simulink model "Sim_Forcing_003h_expe_infra2"  (Simulink 7.4)
settings: Solver=FixedStepDiscrete  StartTime=0.0  StopTime=inf  FixedStep=0.004  RelTol=1e-3
undefined symbols (not defined in the file or in its folder): DiscIntNeverNeededParam
libraries: simulink x42, gt_rt_lib x30, xpcutilitieslib x9, xpclib x2, dspswit3 x1
(part 2 of 5)

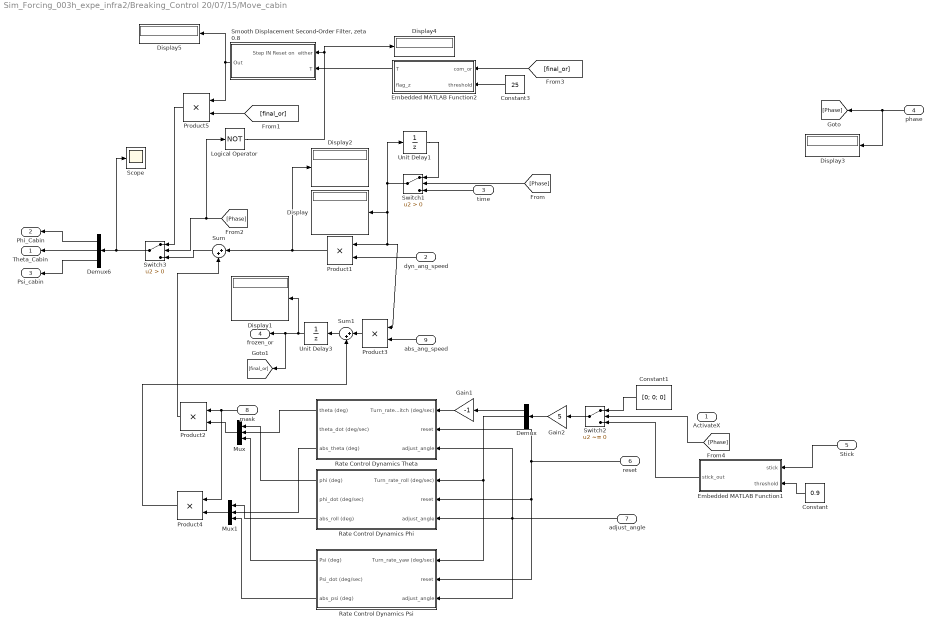
== system Sim_Forcing_003h_expe_infra2/Breaking_Control 20/07/15/Move_cabin ==
  ActivateX : Inport
  dyn_ang_speed : Inport  Port=2
  time : Inport  Port=3
  phase : Inport  Port=4
  Stick : Inport  Port=5
  reset : Inport  Port=6
  adjust_angle : Inport  Port=7
  mask : Inport  Port=8
  abs_ang_speed : Inport  Port=9
  Constant : Constant  Value=0.9  OutDataType=fixdt(1, 16)  OutScaling=2^0
  Constant1 : Constant  Value=[0; 0; 0]  OutDataType=fixdt(1, 16)  OutScaling=2^0
  Constant3 : Constant  Value=25  OutDataType=fixdt(1, 16)  OutScaling=2^0  SampleTime=-1
  Demux : Demux  Outputs=3
  Demux6 : Demux  Outputs=3
  Display{,1..5} (6 alike) : Display
  Embedded MATLAB Function1 : Stateflow chart
  Embedded MATLAB Function2 : Stateflow chart
  Gain1 : Gain  Gain=-1  ParameterDataType=fixdt(1, 16)  ParameterScaling=2^0  OutDataType=fixdt(1, 16)  OutScaling=2^0
  Gain2 : Gain  Gain=5  ParameterDataType=fixdt(1, 16)  ParameterScaling=2^0  OutDataType=fixdt(1, 16)  OutScaling=2^0
  Logical Operator : Logic  Operator=NOT  AllPortsSameDT=off  OutDataTypeMode=boolean  LogicDataType=fixdt(0, 8)  OutDataTypeStr=boolean
  Mux : Mux  Inputs=3
  Mux1 : Mux  Inputs=3
  Product{1..5} (5 alike) : Product  OutDataType=fixdt(1, 16)  OutScaling=2^0  RndMeth=Zero
  Rate Control Dynamics Phi : Subsystem
  Rate Control Dynamics Psi : Subsystem
  Rate Control Dynamics Theta : Subsystem
  Scope : Scope
      settings: TimeRange=10  YMin=0  YMax=4.5e-033  SaveName=ScopeData2
  "Smooth Displacement Second-Order Filter, zeta 0.8" : Subsystem
  Sum : Sum  Inputs=|++  OutDataType=fixdt(1, 16)  OutScaling=2^0
  Sum1 : Sum  Inputs=|++  OutDataType=fixdt(1, 16)  OutScaling=2^0
  Switch1 : Switch  Criteria=u2 > Threshold  OutDataType=fixdt(1, 16)  OutScaling=2^0
  Switch2 : Switch  Criteria=u2 ~= 0  OutDataType=fixdt(1, 16)  OutScaling=2^0
  Switch3 : Switch  Criteria=u2 > Threshold  OutDataType=fixdt(1, 16)  OutScaling=2^0
  Unit Delay1 : UnitDelay  X0=[0 0 0]  SampleTime=-1
  Unit Delay3 : UnitDelay  X0=[0 0 0]  SampleTime=-1
  Theta_Cabin : Outport
  Phi_Cabin : Outport  Port=2
  Psi_cabin : Outport  Port=3
  frozen_or : Outport  Port=4
  wires:
  Demux6/3 -> Psi_cabin/1
  Switch1/1 -> Unit Delay1/1, Display/1, Product1/1, Product3/1
  time/1 -> Switch1/3
  Unit Delay1/1 -> Switch1/1
  Gain2/1 -> Demux/1
  Demux/1 -> Gain1/1
  Demux/2 -> Rate Control Dynamics Phi/1(Turn_rate_roll (deg/sec)), Rate Control Dynamics Psi/1(Turn_rate_yaw (deg/sec))
  Product1/1 -> Display2/1, Sum/1
  reset/1 -> Rate Control Dynamics Theta/2(reset), Rate Control Dynamics Phi/2(reset), Rate Control Dynamics Psi/2(reset)
  adjust_angle/1 -> Rate Control Dynamics Phi/3(adjust_angle), Rate Control Dynamics Theta/3(adjust_angle), Rate Control Dynamics Psi/3(adjust_angle)
  Rate Control Dynamics Theta/1(theta (deg)) -> Mux/2
  Rate Control Dynamics Phi/1(phi (deg)) -> Mux/1
  Mux/1 -> Product2/2
  mask/1 -> Product2/1, Product4/1
  Demux6/1 -> Phi_Cabin/1
  Demux6/2 -> Theta_Cabin/1
  Gain1/1 -> Rate Control Dynamics Theta/1(Turn_rate_pitch (deg/sec))
  Switch2/1 -> Gain2/1
  Rate Control Dynamics Psi/1(Psi (deg)) -> Mux/3
  dyn_ang_speed/1 -> Product1/2
  phase/1 -> [Phase], Display3/1
  [Phase] -> Switch1/2
  Product2/1 -> Sum/2
  Unit Delay3/1 -> Display1/1, frozen_or/1, [final_or]
  Sum1/1 -> Unit Delay3/1
  Product3/1 -> Sum1/1
  abs_ang_speed/1 -> Product3/2
  Mux1/1 -> Product4/2
  Rate Control Dynamics Theta/3(abs_theta (deg)) -> Mux1/2
  Product4/1 -> Sum1/2
  Rate Control Dynamics Phi/3(abs_roll (deg)) -> Mux1/1
  Rate Control Dynamics Psi/3(abs_psi (deg)) -> Mux1/3
  [final_or] -> Product5/2
  "Smooth Displacement Second-Order Filter, zeta 0.8"/1(Out) -> Product5/1, Display5/1
  Switch3/1 -> Demux6/1, Scope/1
  Sum/1 -> Switch3/3
  Product5/1 -> Switch3/1
  [Phase] -> Switch3/2, Logical Operator/1
  Logical Operator/1 -> "Smooth Displacement Second-Order Filter, zeta 0.8"/1(Step IN Reset on  either), Display4/1
  Constant3/1 -> Embedded MATLAB Function2/2(threshold)
  [final_or] -> Embedded MATLAB Function2/1(com_or)
  Embedded MATLAB Function2/1(T) -> "Smooth Displacement Second-Order Filter, zeta 0.8"/2(T)
  Stick/1 -> Embedded MATLAB Function1/1(stick)
  Constant/1 -> Embedded MATLAB Function1/2(threshold)
  [Phase] -> Switch2/2
  Constant1/1 -> Switch2/1
  Embedded MATLAB Function1/1(stick_out) -> Switch2/3

== system Sim_Forcing_003h_expe_infra2/Breaking_Control 20/07/15/Save_data1 ==
  note: we take delay_in + delay_out. We assume it remains cst
  count : Inport  OutDataType=fixdt(1, 16)  OutScaling=2^0
  delay : Inport  Port=2  OutDataType=fixdt(1, 16)  OutScaling=2^0
  Actual_orientation : Inport  Port=3  OutDataType=fixdt(1, 16)  OutScaling=2^0
  com_orientation : Inport  Port=4  OutDataType=fixdt(1, 16)  OutScaling=2^0
  target_ang_speed : Inport  Port=5  OutDataType=fixdt(1, 16)  OutScaling=2^0
  time : Inport  Port=6  OutDataType=fixdt(1, 16)  OutScaling=2^0
  IsinRestPhase : Inport  Port=7  OutDataType=fixdt(1, 16)  OutScaling=2^0
  vis_cond : Inport  Port=8  OutDataType=fixdt(1, 16)  OutScaling=2^0
  Enable : EnablePort  ShowOutputPort=on
  6_DOF Visual Cab 12/06/15 : Subsystem
  Gain : Gain  ParameterDataType=fixdt(1, 16)  ParameterScaling=2^0  OutDataType=fixdt(1, 16)  OutScaling=2^0
  act_or : Display
  or : Display
  wires:
  delay/1 -> Gain/1
  com_orientation/1 -> or/1, 6_DOF Visual Cab 12/06/15/2(Com_or)
  count/1 -> [Cnt]
  time/1 -> [time]
  [time] -> 6_DOF Visual Cab 12/06/15/1(time)
  [targ_ang_speed] -> 6_DOF Visual Cab 12/06/15/5(targ_ang_speed)
  Gain/1 -> 6_DOF Visual Cab 12/06/15/6(delay)
  [reset] -> 6_DOF Visual Cab 12/06/15/8(reset)
  IsinRestPhase/1 -> [RestPhase]
  [RestPhase] -> 6_DOF Visual Cab 12/06/15/7(IsinRestPhase2)
  [Cnt] -> 6_DOF Visual Cab 12/06/15/4(cnt)
  vis_cond/1 -> 6_DOF Visual Cab 12/06/15/3(Vis_cond)
  target_ang_speed/1 -> [targ_ang_speed]
  Actual_orientation/1 -> 6_DOF Visual Cab 12/06/15/9(act_or), act_or/1

== system Sim_Forcing_003h_expe_infra2/Breaking_Control 20/07/15/Send_to_noise_node ==
  note: Send to beat node
  trigger_noise : Inport
  "Byte Packing " : xpcutilitieslib/Byte Packing   MaskPackedDataType=uint8  MaskUnpackedDataTypes={'single'}  MaskAlignment=1
  Constant2 : Constant  Value=9350  OutDataTypeMode=uint16  OutDataType=fixdt(1, 16)  OutScaling=2^0  OutDataTypeStr=uint16
  Constant3 : Constant  Value=4  OutDataTypeMode=uint32  OutDataType=fixdt(1, 16)  OutScaling=2^0  OutDataTypeStr=uint32
  Data Type Conversion : DataTypeConversion  OutDataTypeMode=single  OutDataType=fixdt(1, 16)  OutScaling=2^0  OutDataTypeStr=single
  Display : Display
  GT-RT UDP  Write : gt_rt_lib/GT-RT UDP  Controller  uri='gtp://localhost/udp?port=9350'
  GT-RT UDP TX : gt_rt_lib/GT-RT UDP TX  uri='gtp://localhost/udp?port=9350'  hostname='192.168.102.75'
  Write Error : Display
  wires:
  Constant2/1 -> GT-RT UDP TX/2
  GT-RT UDP TX/1 -> Write Error/1
  Data Type Conversion/1 -> "Byte Packing "/1
  trigger_noise/1 -> Data Type Conversion/1, Display/1
  Constant3/1 -> GT-RT UDP TX/4
  "Byte Packing "/1 -> GT-RT UDP TX/3

== system Sim_Forcing_003h_expe_infra2/Breaking_Control 20/07/15/Smooth Displacement Second-Order Filter, zeta 0.8 ==
  Step IN Reset on  either : Inport
  T : Inport  Port=2  OutDataType=fixdt(1, 16)  OutScaling=2^0
  (zeta*T_transfer)/pi : Gain  Gain=0.8/pi  ParameterDataType=fixdt(1, 16)  ParameterScaling=2^0  OutDataType=fixdt(1, 16)  OutScaling=2^0
  4*zeta*pi : Gain  Gain=3.2*pi  ParameterDataType=fixdt(1, 16)  ParameterScaling=2^0  OutDataType=fixdt(1, 16)  OutScaling=2^0
  4*zeta*pi/T_transfer /s : DiscreteIntegrator  gainval=1  ExternalReset=either  InitialConditionSource=external  SampleTime=0.004  OutDataType=fixdt(1, 16)  OutScaling=2^0  ICPrevOutput=DiscIntNeverNeededParam  ICPrevScaledInput=DiscIntNeverNeededParam
  Discrete Derivative : simulink/Discrete/Discrete Derivative  SystemSampleTime=-1  gainval=1.0  ICPrevScaledInput=0.0  OutMin=[]  OutMax=[]  OutDataType=fixdt(1, 16)  OutScaling=2^-10  DoSatur=off
  Divide : Product  Inputs=*/  OutDataType=fixdt(1, 16)  OutScaling=2^-10
  Divide1 : Product  Inputs=*/  OutDataType=fixdt(1, 16)  OutScaling=2^-10
  For saving position  and velocity until after switchover : UnitDelay  SampleTime=-1
  Product : Product  OutDataType=fixdt(1, 16)  OutScaling=2^0  RndMeth=Zero
  Sum1 : Sum  Inputs=|+-  OutDataType=fixdt(1, 16)  OutScaling=2^0
  Sum2 : Sum  Inputs=-+|  OutDataType=fixdt(1, 16)  OutScaling=2^0
  pi/(zeta*T_transfer)/s : DiscreteIntegrator  gainval=1  ExternalReset=either  InitialConditionSource=external  SampleTime=0.004  OutDataType=fixdt(1, 16)  OutScaling=2^0  ICPrevOutput=DiscIntNeverNeededParam  ICPrevScaledInput=DiscIntNeverNeededParam
  pi/zeta : Gain  Gain=pi/0.8  ParameterDataType=fixdt(1, 16)  ParameterScaling=2^0  OutDataType=fixdt(1, 16)  OutScaling=2^0
  Out : Outport
  wires:
  Discrete Derivative/1 -> Product/2
  Product/1 -> (zeta*T_transfer)/pi/1
  Divide/1 -> 4*zeta*pi/1
  Divide1/1 -> pi/zeta/1
  pi/zeta/1 -> pi/(zeta*T_transfer)/s/1
  pi/(zeta*T_transfer)/s/1 -> Sum2/1, Out/1, For saving position  and velocity until after switchover/1
  4*zeta*pi/T_transfer /s/1 -> Divide1/1, Sum1/2
  Sum1/1 -> Divide/1
  4*zeta*pi/1 -> 4*zeta*pi/T_transfer /s/1
  T/1 -> [T]
  Step IN Reset on  either/1 -> [Step], Sum2/2
  [Step] -> 4*zeta*pi/T_transfer /s/2
  [Step] -> pi/(zeta*T_transfer)/s/2
  [T] -> Divide/2
  For saving position  and velocity until after switchover/1 -> Discrete Derivative/1, pi/(zeta*T_transfer)/s/3
  [T] -> Product/1
  (zeta*T_transfer)/pi/1 -> 4*zeta*pi/T_transfer /s/3
  [T] -> Divide1/2
  Sum2/1 -> Sum1/1

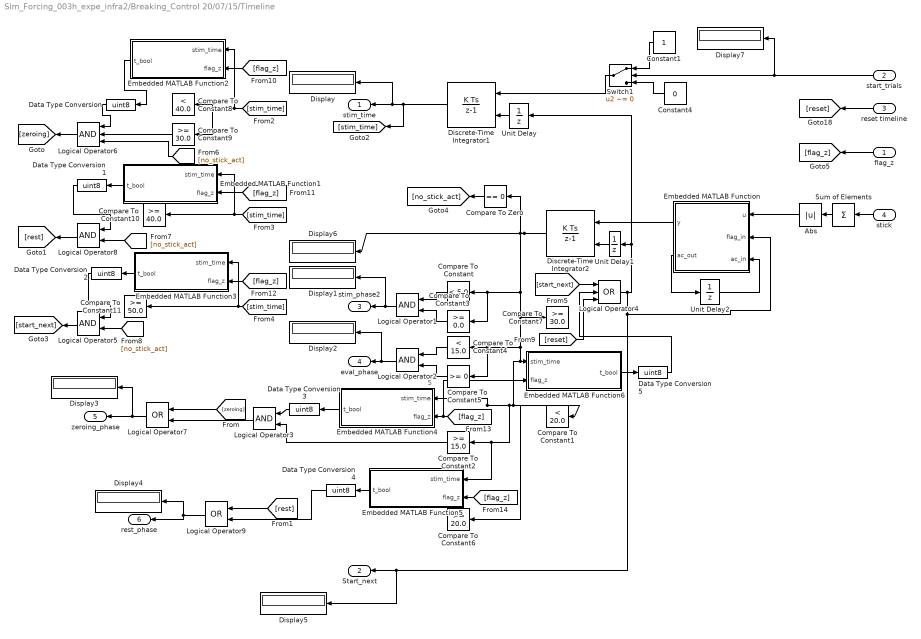
== system Sim_Forcing_003h_expe_infra2/Breaking_Control 20/07/15/Timeline ==
  note: 5
  flag_z : Inport  PortDimensions=1
  start_trials : Inport  Port=2  PortDimensions=1
  reset timeline : Inport  Port=3  PortDimensions=1
  stick : Inport  Port=4
  Abs : Abs  OutDataType=fixdt(1, 16)  OutScaling=2^0
  Compare To Constant : simulink/Logic and Bit Operations/Compare To Constant  SystemSampleTime=-1  relop=<  const=5.0  LogicOutDataTypeMode=uint8
  Compare To Constant1 : simulink/Logic and Bit Operations/Compare To Constant  SystemSampleTime=-1  relop=<  const=20.0  LogicOutDataTypeMode=uint8
  Compare To Constant10 : simulink/Logic and Bit Operations/Compare To Constant  SystemSampleTime=-1  relop=>=  const=40.0  LogicOutDataTypeMode=uint8
  Compare To Constant11 : simulink/Logic and Bit Operations/Compare To Constant  SystemSampleTime=-1  relop=>=  const=50.0  LogicOutDataTypeMode=uint8
  Compare To Constant2 : simulink/Logic and Bit Operations/Compare To Constant  SystemSampleTime=-1  relop=>=  const=15.0  LogicOutDataTypeMode=uint8
  Compare To Constant3 : simulink/Logic and Bit Operations/Compare To Constant  SystemSampleTime=-1  relop=>=  const=0.0  LogicOutDataTypeMode=uint8
  Compare To Constant4 : simulink/Logic and Bit Operations/Compare To Constant  SystemSampleTime=-1  relop=<  const=15.0  LogicOutDataTypeMode=uint8
  Compare To Constant5 : simulink/Logic and Bit Operations/Compare To Constant  SystemSampleTime=-1  relop=>=  const=0  LogicOutDataTypeMode=uint8
  Compare To Constant6 : simulink/Logic and Bit Operations/Compare To Constant  SystemSampleTime=-1  relop=>=  const=20.0  LogicOutDataTypeMode=uint8
  Compare To Constant7 : simulink/Logic and Bit Operations/Compare To Constant  SystemSampleTime=-1  relop=>=  const=30.0  LogicOutDataTypeMode=uint8
  Compare To Constant8 : simulink/Logic and Bit Operations/Compare To Constant  SystemSampleTime=-1  relop=<  const=40.0  LogicOutDataTypeMode=uint8
  Compare To Constant9 : simulink/Logic and Bit Operations/Compare To Constant  SystemSampleTime=-1  relop=>=  const=30.0  LogicOutDataTypeMode=uint8
  Compare To Zero : simulink/Logic and Bit Operations/Compare To Zero  SystemSampleTime=-1  relop===  LogicOutDataTypeMode=uint8
  Constant1 : Constant  OutDataType=fixdt(1, 16)  OutScaling=2^0
  Constant4 : Constant  Value=0  OutDataType=fixdt(1, 16)  OutScaling=2^0
  Data Type Conversion{,1..5} (6 alike) : DataTypeConversion  OutDataTypeMode=uint8  OutDataType=fixdt(1, 16)  OutScaling=2^0  OutDataTypeStr=uint8
  Discrete-Time Integrator1 : DiscreteIntegrator  ExternalReset=rising  SampleTime=0.004  LimitOutput=on  UpperSaturationLimit=60  LowerSaturationLimit=0  ICPrevOutput=DiscIntNeverNeededParam  ICPrevScaledInput=DiscIntNeverNeededParam
  Discrete-Time Integrator2 : DiscreteIntegrator  ExternalReset=level  SampleTime=0.004  LimitOutput=on  UpperSaturationLimit=40  LowerSaturationLimit=0  ICPrevOutput=DiscIntNeverNeededParam  ICPrevScaledInput=DiscIntNeverNeededParam
  Display{,1..7} (8 alike) : Display
  Embedded MATLAB Function : Stateflow chart
  Embedded MATLAB Function1 : Stateflow chart
  Embedded MATLAB Function2 : Stateflow chart
  Embedded MATLAB Function3 : Stateflow chart
  Embedded MATLAB Function4 : Stateflow chart
  Embedded MATLAB Function5 : Stateflow chart
  Embedded MATLAB Function6 : Stateflow chart
  Logical Operator{1..3,5,8} (5 alike) : Logic  AllPortsSameDT=off  OutDataTypeMode=boolean  LogicDataType=fixdt(0, 8)  OutDataTypeStr=boolean
  Logical Operator4 : Logic  Operator=OR  Inputs=3  AllPortsSameDT=off  OutDataTypeMode=boolean  LogicDataType=fixdt(0, 8)  OutDataTypeStr=boolean
  Logical Operator6 : Logic  Inputs=3  AllPortsSameDT=off  OutDataTypeMode=boolean  LogicDataType=fixdt(0, 8)  OutDataTypeStr=boolean
  Logical Operator7 : Logic  Operator=OR  AllPortsSameDT=off  OutDataTypeMode=boolean  LogicDataType=fixdt(0, 8)  OutDataTypeStr=boolean
  Logical Operator9 : Logic  Operator=OR  AllPortsSameDT=off  OutDataTypeMode=boolean  LogicDataType=fixdt(0, 8)  OutDataTypeStr=boolean
  Sum of Elements : Sum  Inputs=+  OutDataType=fixdt(1, 16)  OutScaling=2^-10
  Switch1 : Switch  Criteria=u2 ~= 0  Threshold=0.2  OutDataType=fixdt(1, 16)  OutScaling=2^0
  Unit Delay : UnitDelay  SampleTime=-1
  Unit Delay1 : UnitDelay  SampleTime=-1
  Unit Delay2 : UnitDelay  SampleTime=-1
  stim_time : Outport  OutDataType=fixdt(1, 16)  OutScaling=2^0
  Start_next : Outport  Port=2  OutDataType=fixdt(1, 16)  OutScaling=2^0
  stim_phase2 : Outport  Port=3  OutDataType=fixdt(1, 16)  OutScaling=2^0
  eval_phase : Outport  Port=4  OutDataType=fixdt(1, 16)  OutScaling=2^0
  zeroing_phase : Outport  Port=5  OutDataType=fixdt(1, 16)  OutScaling=2^0
  rest_phase : Outport  Port=6  OutDataType=fixdt(1, 16)  OutScaling=2^0
  wires:
  Discrete-Time Integrator1/1 -> stim_time/1, Display/1, [stim_time]
  Embedded MATLAB Function/1(y) -> Discrete-Time Integrator2/1
  Discrete-Time Integrator2/1 -> Compare To Constant/1, Compare To Constant3/1, Compare To Constant4/1, Compare To Constant5/1, Compare To Constant1/1, Embedded MATLAB Function4/1(stim_time), Compare To Constant2/1, Embedded MATLAB Function5/1(stim_time), Compare To Constant6/1, Embedded MATLAB Function6/1(stim_time), Compare To Constant7/1, Display6/1, Compare To Zero/1
  Compare To Constant/1 -> Logical Operator1/1
  Compare To Constant3/1 -> Logical Operator1/2
  Logical Operator1/1 -> stim_phase2/1, Display1/1
  Compare To Constant4/1 -> Logical Operator2/1
  Compare To Constant5/1 -> Logical Operator2/2
  Logical Operator2/1 -> eval_phase/1, Display2/1
  Compare To Constant2/1 -> Logical Operator3/2
  Logical Operator3/1 -> Logical Operator7/2
  Logical Operator4/1 -> Start_next/1, Display5/1, Embedded MATLAB Function/2(flag_in), Unit Delay1/1, Unit Delay/1
  Constant1/1 -> Switch1/1
  Switch1/1 -> Discrete-Time Integrator1/1
  start_trials/1 -> Switch1/2, Display7/1
  Constant4/1 -> Switch1/3
  stick/1 -> Sum of Elements/1
  Unit Delay/1 -> Discrete-Time Integrator1/2
  Unit Delay1/1 -> Discrete-Time Integrator2/2
  Sum of Elements/1 -> Abs/1
  Abs/1 -> Embedded MATLAB Function/1(u)
  Embedded MATLAB Function/2(ac_out) -> Unit Delay2/1
  Unit Delay2/1 -> Embedded MATLAB Function/3(ac_in)
  Compare To Constant9/1 -> Logical Operator6/2
  Logical Operator7/1 -> zeroing_phase/1, Display3/1
  Logical Operator9/1 -> rest_phase/1, Display4/1
  Logical Operator6/1 -> [zeroing]
  [zeroing] -> Logical Operator7/1
  Logical Operator8/1 -> [rest]
  [rest] -> Logical Operator9/1
  [stim_time] -> Compare To Constant8/1, Compare To Constant9/1, Embedded MATLAB Function2/1(stim_time)
  [stim_time] -> Compare To Constant10/1, Embedded MATLAB Function1/1(stim_time)
  [stim_time] -> Compare To Constant11/1, Embedded MATLAB Function3/1(stim_time)
  Logical Operator5/1 -> [start_next]
  [start_next] -> Logical Operator4/1
  Compare To Zero/1 -> [no_stick_act]
  [no_stick_act] -> Logical Operator6/3
  [no_stick_act] -> Logical Operator8/2
  [no_stick_act] -> Logical Operator5/2
  reset timeline/1 -> [reset]
  [reset] -> Logical Operator4/3
  flag_z/1 -> [flag_z]
  [flag_z] -> Embedded MATLAB Function2/2(flag_z)
  [flag_z] -> Embedded MATLAB Function1/2(flag_z)
  [flag_z] -> Embedded MATLAB Function3/2(flag_z)
  [flag_z] -> Embedded MATLAB Function4/2(flag_z), Embedded MATLAB Function6/2(flag_z)
  [flag_z] -> Embedded MATLAB Function5/2(flag_z)
  Embedded MATLAB Function2/1(t_bool) -> Data Type Conversion/1
  Data Type Conversion/1 -> Logical Operator6/1
  Embedded MATLAB Function1/1(t_bool) -> Data Type Conversion1/1
  Data Type Conversion1/1 -> Logical Operator8/1
  Embedded MATLAB Function3/1(t_bool) -> Data Type Conversion2/1
  Data Type Conversion2/1 -> Logical Operator5/1
  Embedded MATLAB Function4/1(t_bool) -> Data Type Conversion3/1
  Data Type Conversion3/1 -> Logical Operator3/1
  Embedded MATLAB Function5/1(t_bool) -> Data Type Conversion4/1
  Data Type Conversion4/1 -> Logical Operator9/2
  Embedded MATLAB Function6/1(t_bool) -> Data Type Conversion5/1
  Data Type Conversion5/1 -> Logical Operator4/2

== system Sim_Forcing_003h_expe_infra2/Breaking_Control 20/07/15/select_ang_speed ==
  Count : Inport  OutDataType=fixdt(1, 16)  OutScaling=2^0
  eval_phase : Inport  Port=2  OutDataType=fixdt(1, 16)  OutScaling=2^0
  Constant : Constant  Value=[0 0 0]  OutDataType=fixdt(1, 16)  OutScaling=2^0
  Embedded MATLAB Function2 : Stateflow chart
  Switch : Switch  Criteria=u2 ~= 0  OutDataType=fixdt(1, 16)  OutScaling=2^0
  Unit Delay : UnitDelay  SampleTime=-1
  Target_ang_speed : Outport
  mask : Outport  Port=2
  vis_cond : Outport  Port=3
  flag_out : Outport  Port=4
  wires:
  Count/1 -> Embedded MATLAB Function2/1(count)
  eval_phase/1 -> Switch/2
  Embedded MATLAB Function2/1(target_ang_speed) -> Switch/3, Target_ang_speed/1
  Constant/1 -> Switch/1
  Embedded MATLAB Function2/2(mask) -> mask/1
  Embedded MATLAB Function2/3(vis_cond) -> vis_cond/1
  Embedded MATLAB Function2/4(flag_out) -> flag_out/1
  Embedded MATLAB Function2/5(endOffile_out) -> Unit Delay/1
  Unit Delay/1 -> Embedded MATLAB Function2/2(endOffile_in)

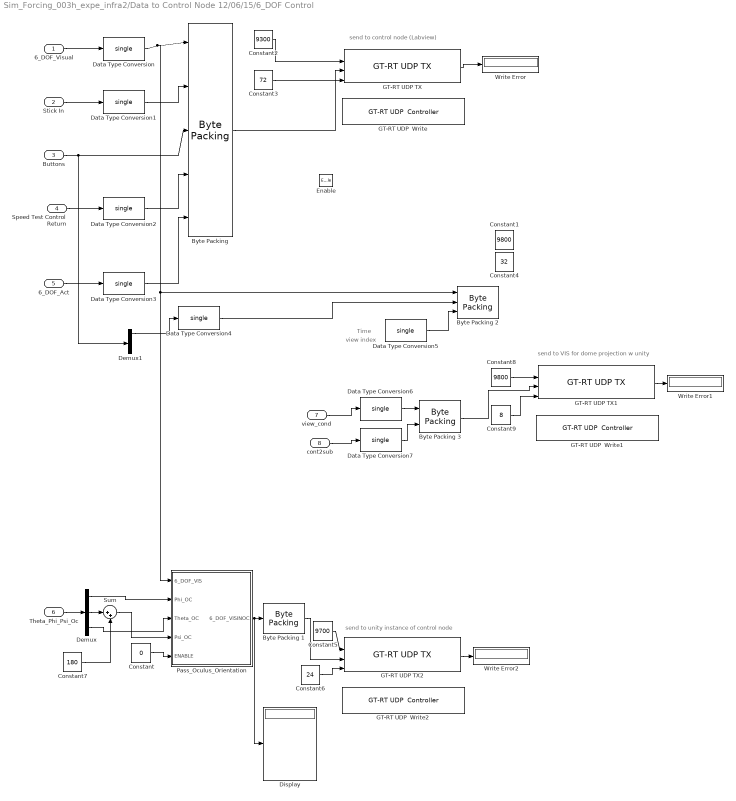
== system Sim_Forcing_003h_expe_infra2/Data to Control Node 12/06/15/6_DOF Control ==
  note: send to control node (Labview)
  note: send to unity instance of control node
  note: send to VIS for dome projection w unity
  note: Time
  note: view index
  6_DOF_Visual : Inport
  Stick In : Inport  Port=2
  Buttons : Inport  Port=3
  Speed Test Control Return : Inport  Port=4
  6_DOF_Act : Inport  Port=5
  Theta_Phi_Psi_Oc : Inport  Port=6
  view_cond : Inport  Port=7
  cont2sub : Inport  Port=8
  Enable : EnablePort
  Byte Packing {,1..3} (4 alike) : xpcutilitieslib/Byte Packing 
  Constant : Constant  Value=0  OutDataType=fixdt(1, 16)  OutScaling=2^0
  Constant1 : Constant  Value=9800  OutDataTypeMode=uint16  OutDataType=fixdt(1, 16)  OutScaling=2^0  OutDataTypeStr=uint16
  Constant2 : Constant  Value=9300  OutDataTypeMode=uint16  OutDataType=fixdt(1, 16)  OutScaling=2^0  OutDataTypeStr=uint16
  Constant3 : Constant  Value=72  OutDataTypeMode=uint32  OutDataType=fixdt(1, 16)  OutScaling=2^0  OutDataTypeStr=uint32
  Constant4 : Constant  Value=32  OutDataTypeMode=uint32  OutDataType=fixdt(1, 16)  OutScaling=2^0  OutDataTypeStr=uint32
  Constant5 : Constant  Value=9700  OutDataTypeMode=uint16  OutDataType=fixdt(1, 16)  OutScaling=2^0  OutDataTypeStr=uint16
  Constant6 : Constant  Value=24  OutDataTypeMode=uint32  OutDataType=fixdt(1, 16)  OutScaling=2^0  OutDataTypeStr=uint32
  Constant7 : Constant  Value=180  OutDataType=fixdt(1, 16)  OutScaling=2^0
  Constant8 : Constant  Value=9800  OutDataTypeMode=uint16  OutDataType=fixdt(1, 16)  OutScaling=2^0  OutDataTypeStr=uint16
  Constant9 : Constant  Value=8  OutDataTypeMode=uint32  OutDataType=fixdt(1, 16)  OutScaling=2^0  OutDataTypeStr=uint32
  Data Type Conversion{,1..7} (8 alike) : DataTypeConversion  OutDataTypeMode=single  OutDataType=fixdt(1, 16)  OutScaling=2^0  OutDataTypeStr=single
  Demux : Demux  Outputs=3
  Demux1 : Demux  Outputs=8
  Display : Display
  GT-RT UDP  Write : gt_rt_lib/GT-RT UDP  Controller  uri='gtp://localhost/udp?port=9300'
  GT-RT UDP  Write1 : gt_rt_lib/GT-RT UDP  Controller  uri='gtp://localhost/udp?port=9800'
  GT-RT UDP  Write2 : gt_rt_lib/GT-RT UDP  Controller  uri='gtp://localhost/udp?port=9700'
  GT-RT UDP TX : gt_rt_lib/GT-RT UDP TX  uri='gtp://localhost/udp?port=9300'  hostname='192.168.102.75'
  GT-RT UDP TX1 : gt_rt_lib/GT-RT UDP TX  uri='gtp://localhost/udp?port=9800'  hostname='192.168.102.13'
  GT-RT UDP TX2 : gt_rt_lib/GT-RT UDP TX  uri='gtp://localhost/udp?port=9700'  hostname='192.168.102.75'
  Pass_Oculus_Orientation : Subsystem
  Sum : Sum  Inputs=|++  OutDataType=fixdt(1, 16)  OutScaling=2^0
  Write Error : Display
  Write Error1 : Display
  Write Error2 : Display
  wires:
  Constant2/1 -> GT-RT UDP TX/2
  Constant3/1 -> GT-RT UDP TX/4
  GT-RT UDP TX/1 -> Write Error/1
  Data Type Conversion/1 -> "Byte Packing "/1, Pass_Oculus_Orientation/1(6_DOF_VIS), Byte Packing 2/1
  "Byte Packing "/1 -> GT-RT UDP TX/3
  Stick In/1 -> Data Type Conversion1/1
  Data Type Conversion1/1 -> "Byte Packing "/2
  Buttons/1 -> "Byte Packing "/3, Demux1/1
  Speed Test Control Return/1 -> Data Type Conversion2/1
  Data Type Conversion2/1 -> "Byte Packing "/4
  6_DOF_Act/1 -> Data Type Conversion3/1
  Data Type Conversion3/1 -> "Byte Packing "/5
  GT-RT UDP TX1/1 -> Write Error1/1
  GT-RT UDP TX2/1 -> Write Error2/1
  Constant5/1 -> GT-RT UDP TX2/2
  Constant6/1 -> GT-RT UDP TX2/4
  Pass_Oculus_Orientation/1(6_DOF_VISINOC) -> Byte Packing 1/1, Display/1
  Constant/1 -> Pass_Oculus_Orientation/5(ENABLE)
  Byte Packing 1/1 -> GT-RT UDP TX2/3
  Theta_Phi_Psi_Oc/1 -> Demux/1
  Demux/2 -> Sum/1
  Sum/1 -> Pass_Oculus_Orientation/4(Psi_OC)
  Constant7/1 -> Sum/2
  Demux/1 -> Pass_Oculus_Orientation/2(Phi_OC)
  Demux/3 -> Pass_Oculus_Orientation/3(Theta_OC)
  Data Type Conversion4/1 -> Byte Packing 2/2
  Data Type Conversion5/1 -> Byte Packing 2/3
  Demux1/2 -> Data Type Conversion4/1
  6_DOF_Visual/1 -> Data Type Conversion/1
  Constant8/1 -> GT-RT UDP TX1/2
  Constant9/1 -> GT-RT UDP TX1/4
  Byte Packing 3/1 -> GT-RT UDP TX1/3
  view_cond/1 -> Data Type Conversion6/1
  Data Type Conversion6/1 -> Byte Packing 3/1
  cont2sub/1 -> Data Type Conversion7/1
  Data Type Conversion7/1 -> Byte Packing 3/2

== system Sim_Forcing_003h_expe_infra2/Data to Control Node 12/06/15/Interaction device from VIS (Stick)  ==
  Display2 : Display
  Display4 : Display
  Display5 : Display
  Error : Display
  GT-RT UDP  Read : gt_rt_lib/GT-RT UDP  Controller  uri='gtp://localhost/udp?port=9600'
  GT-RT UDP RX : gt_rt_lib/GT-RT UDP RX  uri='gtp://localhost/udp?port=9600'  receive_buffer_size=28  timeout=0  sample_time=0.004
  Terminator : Terminator
  Unpack : xpclib/UDP/Unpack  dimensions={3,8,1,1}  datatypes={'single','uint8','single','single'}  byteAlign=1
  Stick Out : Outport  OutDataType=fixdt(1, 16)  OutScaling=2^0
  Buttons : Outport  Port=2  OutDataType=fixdt(1, 16)  OutScaling=2^0
  Speed_Test_VIS_Send : Outport  Port=3  OutDataType=fixdt(1, 16)  OutScaling=2^0
  for_delay_calc : Outport  Port=4  OutDataType=fixdt(1, 16)  OutScaling=2^0
  wires:
  GT-RT UDP RX/2 -> Display2/1
  GT-RT UDP RX/6 -> Error/1
  GT-RT UDP RX/5 -> Display4/1
  GT-RT UDP RX/4 -> Display5/1
  GT-RT UDP RX/1 -> Unpack/1
  GT-RT UDP RX/3 -> Terminator/1
  Unpack/1 -> Stick Out/1
  Unpack/2 -> Buttons/1
  Unpack/3 -> Speed_Test_VIS_Send/1
  Unpack/4 -> for_delay_calc/1

== system Sim_Forcing_003h_expe_infra2/Handshake CAN/If Action Subsystem ==
  Action Port : ActionPort
  GT-RT CAN TX : gt_rt_lib/GT-RT CAN TX  uri='gt_rt_dev://localhost/dev/can0#0'  mff=MFF_11_DAT
  TX CAN ID1 : Constant  Value=hex2dec('100')  OutDataTypeMode=uint32  OutDataType=sfix(16)  OutScaling=2^0  OutDataTypeStr=uint32
  TX Data : Constant  OutDataTypeMode=uint8  OutDataType=sfix(16)  OutScaling=2^0  OutDataTypeStr=uint8
  wires:
  TX CAN ID1/1 -> GT-RT CAN TX/1
  TX Data/1 -> GT-RT CAN TX/2

== system Sim_Forcing_003h_expe_infra2/Handshake CAN/If Action Subsystem1 ==
  Action Port : ActionPort  ActionType=then
  GT-RT CAN TX : gt_rt_lib/GT-RT CAN TX  uri='gt_rt_dev://localhost/dev/can0#0'  mff=MFF_11_DAT
  TX CAN ID1 : Constant  Value=hex2dec('100')  OutDataTypeMode=uint32  OutDataType=sfix(16)  OutScaling=2^0  OutDataTypeStr=uint32
  TX Data : Constant  OutDataTypeMode=uint8  OutDataType=sfix(16)  OutScaling=2^0  OutDataTypeStr=uint8
  wires:
  TX CAN ID1/1 -> GT-RT CAN TX/1
  TX Data/1 -> GT-RT CAN TX/2

== system Sim_Forcing_003h_expe_infra2/Joint Controller (May 7, 2015)/Forward Kinematics ==
  J_ANG_ACT : Inport
  Data Type Conversion4 : DataTypeConversion  OutDataTypeMode=double  OutDataType=fixdt(1, 16)  OutScaling=2^0  OutDataTypeStr=double
  Demux1 : Demux  Outputs=[3,1,1,1]
  Embedded MATLAB Function : Stateflow chart
  KUKA2NED : Subsystem
  Mux : Mux  Inputs=2
  6-DOF_ACT : Outport
  roll_pitch_act : Outport  Port=2
  wires:
  KUKA2NED/1(NED) -> Embedded MATLAB Function/1(vec)
  Embedded MATLAB Function/1(out) -> 6-DOF_ACT/1, Data Type Conversion4/1
  J_ANG_ACT/1 -> KUKA2NED/1(KUKA)
  Demux1/3 -> Mux/2
  Demux1/2 -> Mux/1
  Mux/1 -> roll_pitch_act/1
  Data Type Conversion4/1 -> Demux1/1

== system Sim_Forcing_003h_expe_infra2/Joint Controller (May 7, 2015)/Increments ==
  J_ANG : Inport
  Sum6 : Sum  Inputs=|+-  OutDataType=fixdt(1, 16)  OutScaling=2^0
  Unit Delay6 : UnitDelay  X0=[0 50 -68 0 18 0]'  SampleTime=-1
  J_ANG_INC : Outport
  wires:
  Unit Delay6/1 -> Sum6/2
  J_ANG/1 -> Unit Delay6/1, Sum6/1
  Sum6/1 -> J_ANG_INC/1

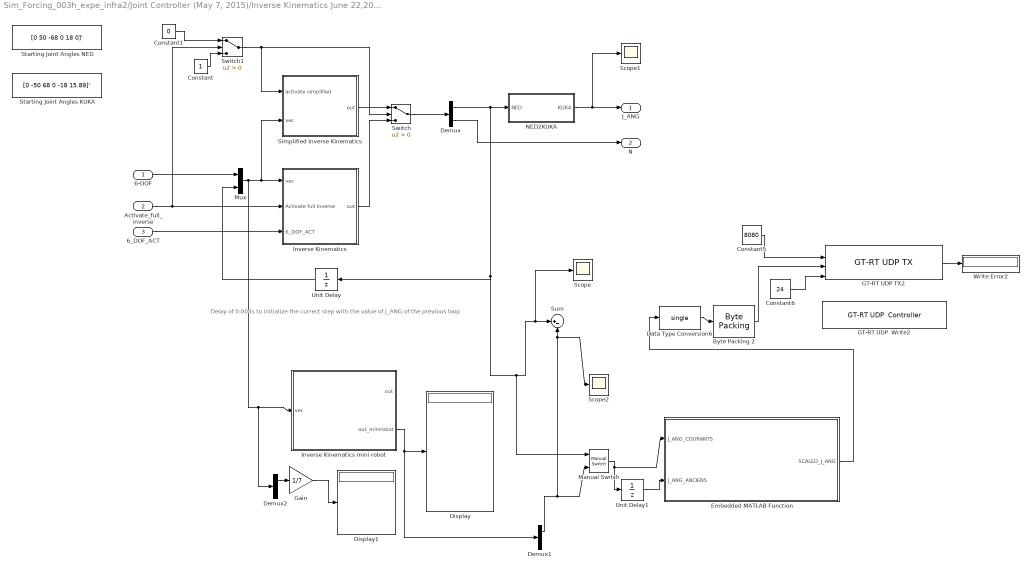
== system Sim_Forcing_003h_expe_infra2/Joint Controller (May 7, 2015)/Inverse Kinematics June 22,2016 compatible_minirobot ==
  note: Delay of 0.004s to initialize the currect step with the value of J_ANG of the previous loop
  6-DOF : Inport  OutDataType=fixdt(1, 16)  OutScaling=2^0
  Activate_full_inverse : Inport  Port=2  OutDataType=fixdt(1, 16)  OutScaling=2^0
  6_DOF_ACT : Inport  Port=3  OutDataType=fixdt(1, 16)  OutScaling=2^0
  Byte Packing 2 : xpcutilitieslib/Byte Packing   MaskPackedDataType=uint8  MaskUnpackedDataTypes={'single'}  MaskAlignment=1
  Constant : Constant  OutDataType=fixdt(1, 16)  OutScaling=2^0
  Constant1 : Constant  Value=0  OutDataType=fixdt(1, 16)  OutScaling=2^0
  Constant5 : Constant  Value=8080  OutDataTypeMode=uint16  OutDataType=fixdt(1, 16)  OutScaling=2^0  OutDataTypeStr=uint16
  Constant6 : Constant  Value=24  OutDataTypeMode=uint32  OutDataType=fixdt(1, 16)  OutScaling=2^0  OutDataTypeStr=uint32
  Data Type Conversion6 : DataTypeConversion  OutDataTypeMode=single  OutDataType=fixdt(1, 16)  OutScaling=2^0  OutDataTypeStr=single
  Demux : Demux  Outputs=[6 1]
  Demux1 : Demux  Outputs=[6 1]
  Demux2 : Demux  Outputs=[3,9]
  Display : Display
  Display1 : Display
  Embedded MATLAB Function : Stateflow chart
  GT-RT UDP  Write2 : gt_rt_lib/GT-RT UDP  Controller  uri='gtp://localhost/udp?port=8080'
  GT-RT UDP TX2 : gt_rt_lib/GT-RT UDP TX  uri='gtp://localhost/udp?port=8080'  hostname='192.168.102.76'
  Gain : Gain  Gain=1/7  ParameterDataType=fixdt(1, 16)  ParameterScaling=2^0  OutDataType=fixdt(1, 16)  OutScaling=2^0
  Inverse Kinematics : Subsystem
  Inverse Kinematics mini robot : Subsystem
  Manual Switch : simulink/Signal Routing/Manual Switch  SystemSampleTime=-1  sw=0  action=0  varsize=off
  Mux : Mux  Inputs=2
  NED2KUKA : Subsystem
  Scope : Scope
      settings: TimeRange=10  YMin=-70  YMax=110
  Scope1 : Scope
      settings: YMin=-90  YMax=130  SaveName=ScopeData4
  Scope2 : Scope
      settings: YMin=-70  YMax=110
  Simplified Inverse Kinematics : Subsystem
  Starting Joint Angles KUKA : Constant  Value=[0 -50 68 0 -18 15.89]'  OutDataType=fixdt(1, 16)  OutScaling=2^0
  Starting Joint Angles NED : Constant  Value=[0 50 -68 0 18 0]'  OutDataType=fixdt(1, 16)  OutScaling=2^0
  Sum : Sum  Inputs=|+-  OutDataType=fixdt(1, 16)  OutScaling=2^0
  Switch : Switch  Criteria=u2 > Threshold  OutDataType=fixdt(1, 16)  OutScaling=2^0
  Switch1 : Switch  Criteria=u2 > Threshold  OutDataType=fixdt(1, 16)  OutScaling=2^0
  Unit Delay : UnitDelay  X0=[0 50 -68 0 18 0]'  SampleTime=-1
  Unit Delay1 : UnitDelay  X0=[0 50 -68 0 18 0]'  SampleTime=-1
  Write Error2 : Display
  J_ANG : Outport  OutDataType=fixdt(1, 16)  OutScaling=2^0
  N : Outport  Port=2  OutDataType=fixdt(1, 16)  OutScaling=2^0
  wires:
  NED2KUKA/1(KUKA) -> Scope1/1, J_ANG/1
  6-DOF/1 -> Mux/1
  Unit Delay/1 -> Mux/2
  Demux/1 -> NED2KUKA/1(NED), Unit Delay/1, Manual Switch/1, Sum/1, Scope/1
  Demux/2 -> N/1
  Simplified Inverse Kinematics/1(out) -> Switch/1
  Inverse Kinematics/1(out) -> Switch/3
  Switch/1 -> Demux/1
  Mux/1 -> Inverse Kinematics/1(vec), Simplified Inverse Kinematics/2(vec), Inverse Kinematics mini robot/1(vec), Demux2/1
  Activate_full_inverse/1 -> Inverse Kinematics/2(Activate full inverse), Switch1/2
  Switch1/1 -> Simplified Inverse Kinematics/1(activate simplified), Switch/2
  Constant/1 -> Switch1/3
  6_DOF_ACT/1 -> Inverse Kinematics/3(6_DOF_ACT)
  Constant5/1 -> GT-RT UDP TX2/2
  GT-RT UDP TX2/1 -> Write Error2/1
  Constant6/1 -> GT-RT UDP TX2/4
  Inverse Kinematics mini robot/2(out_minirobot) -> Display/1, Demux1/1
  Byte Packing 2/1 -> GT-RT UDP TX2/3
  Demux2/1 -> Gain/1
  Gain/1 -> Display1/1
  Demux1/1 -> Manual Switch/2, Sum/2, Scope2/1
  Data Type Conversion6/1 -> Byte Packing 2/1
  Constant1/1 -> Switch1/1
  Manual Switch/1 -> Unit Delay1/1, Embedded MATLAB Function/1(J_ANG_COURANTS)
  Unit Delay1/1 -> Embedded MATLAB Function/2(J_ANG_ANCIENS)
  Embedded MATLAB Function/1(SCALED_J_ANG) -> Data Type Conversion6/1

== system Sim_Forcing_003h_expe_infra2/Joint Controller (May 7, 2015)/Inverse Kinematics May 6, 2015 ==
  note: Delay of 0.004s to initialize the currect step with the value of J_ANG of the previous loop
  6-DOF : Inport  OutDataType=fixdt(1, 16)  OutScaling=2^0
  Activate_full_inverse : Inport  Port=2  OutDataType=fixdt(1, 16)  OutScaling=2^0
  6_DOF_ACT : Inport  Port=3  OutDataType=fixdt(1, 16)  OutScaling=2^0
  Constant : Constant  OutDataType=fixdt(1, 16)  OutScaling=2^0
  Demux : Demux  Outputs=[6 1]
  Ground : Ground
  Inverse Kinematics : Subsystem
  Mux : Mux  Inputs=2
  NED2KUKA : Subsystem
  Scope1 : Scope
      settings: YMin=-50  YMax=70  SaveName=ScopeData4
  Simplified Inverse Kinematics : Subsystem
  Starting Joint Angles KUKA : Constant  Value=[0 -50 68 0 -18 15.89]'  OutDataType=fixdt(1, 16)  OutScaling=2^0
  Starting Joint Angles NED : Constant  Value=[0 50 -68 0 18 0]'  OutDataType=fixdt(1, 16)  OutScaling=2^0
  Switch : Switch  Criteria=u2 > Threshold  OutDataType=fixdt(1, 16)  OutScaling=2^0
  Switch1 : Switch  Criteria=u2 > Threshold  OutDataType=fixdt(1, 16)  OutScaling=2^0
  Unit Delay : UnitDelay  X0=[0 50 -68 0 18 0]'  SampleTime=-1
  J_ANG : Outport  OutDataType=fixdt(1, 16)  OutScaling=2^0
  N : Outport  Port=2  OutDataType=fixdt(1, 16)  OutScaling=2^0
  wires:
  NED2KUKA/1(KUKA) -> Scope1/1, J_ANG/1
  6-DOF/1 -> Mux/1
  Unit Delay/1 -> Mux/2
  Demux/1 -> NED2KUKA/1(NED), Unit Delay/1
  Demux/2 -> N/1
  Simplified Inverse Kinematics/1(out) -> Switch/1
  Inverse Kinematics/1(out) -> Switch/3
  Switch/1 -> Demux/1
  Mux/1 -> Inverse Kinematics/1(vec), Simplified Inverse Kinematics/2(vec)
  Activate_full_inverse/1 -> Inverse Kinematics/2(Activate full inverse), Switch1/2
  Ground/1 -> Switch1/1
  Switch1/1 -> Simplified Inverse Kinematics/1(activate simplified), Switch/2
  Constant/1 -> Switch1/3
  6_DOF_ACT/1 -> Inverse Kinematics/3(6_DOF_ACT)

== system Sim_Forcing_003h_expe_infra2/Joint Controller (May 7, 2015)/Subtract psi offset ==
  Psi_Offset : Inport
  J_ANG_ACT : Inport  Port=2
  Data Type Conversion : DataTypeConversion  OutDataTypeMode=double  OutDataType=fixdt(1, 16)  OutScaling=2^0  OutDataTypeStr=double
  Demux1 : Demux  Outputs=[1,5]
  Mux1 : Mux  Inputs=[1,5]
  Sum3 : Sum  Inputs=-+|  OutDataType=fixdt(1, 16)  OutScaling=2^0
  out : Outport
  wires:
  Demux1/1 -> Sum3/2
  Sum3/1 -> Mux1/1
  Demux1/2 -> Mux1/2
  J_ANG_ACT/1 -> Data Type Conversion/1
  Mux1/1 -> out/1
  Data Type Conversion/1 -> Demux1/1
  Psi_Offset/1 -> Sum3/1

== system Sim_Forcing_003h_expe_infra2/BEC (May 7, 2015)/CAN Receive/Convert 4*uni8 to int ==
  byte0 : Inport
  byte1 : Inport  Port=2
  byte2 : Inport  Port=3
  byte3 : Inport  Port=4
  Add : Sum  Inputs=++++  OutDataTypeMode=int32  OutDataType=fixdt(1, 16)  OutScaling=2^-10  OutDataTypeStr=int32
  Gain2 : Gain  Gain=256  ParameterDataType=fixdt(1, 16)  ParameterScaling=2^0  OutDataType=fixdt(1, 16)  OutScaling=2^0
  Gain3 : Gain  Gain=2^16  ParameterDataType=fixdt(1, 16)  ParameterScaling=2^0  OutDataType=fixdt(1, 16)  OutScaling=2^0
  Gain4 : Gain  Gain=2^24  ParameterDataType=fixdt(1, 16)  ParameterScaling=2^0  OutDataType=fixdt(1, 16)  OutScaling=2^0
  int : Outport
  wires:
  Gain2/1 -> Add/2
  Gain3/1 -> Add/3
  byte0/1 -> Add/1
  Add/1 -> int/1
  byte1/1 -> Gain2/1
  byte2/1 -> Gain3/1
  byte3/1 -> Gain4/1
  Gain4/1 -> Add/4

== system Sim_Forcing_003h_expe_infra2/BEC (May 7, 2015)/CAN Receive/Convert 4*uni8 to int1 ==
  byte0 : Inport
  byte1 : Inport  Port=2
  byte2 : Inport  Port=3
  byte3 : Inport  Port=4
  Add : Sum  Inputs=++++  OutDataTypeMode=int32  OutDataType=fixdt(1, 16)  OutScaling=2^-10  OutDataTypeStr=int32
  Gain2 : Gain  Gain=256  ParameterDataType=fixdt(1, 16)  ParameterScaling=2^0  OutDataType=fixdt(1, 16)  OutScaling=2^0
  Gain3 : Gain  Gain=2^16  ParameterDataType=fixdt(1, 16)  ParameterScaling=2^0  OutDataType=fixdt(1, 16)  OutScaling=2^0
  Gain4 : Gain  Gain=2^24  ParameterDataType=fixdt(1, 16)  ParameterScaling=2^0  OutDataType=fixdt(1, 16)  OutScaling=2^0
  int : Outport
  wires:
  Gain4/1 -> Add/4
  byte3/1 -> Gain4/1
  byte2/1 -> Gain3/1
  byte1/1 -> Gain2/1
  Add/1 -> int/1
  byte0/1 -> Add/1
  Gain3/1 -> Add/3
  Gain2/1 -> Add/2

== system Sim_Forcing_003h_expe_infra2/BEC (May 7, 2015)/CAN Receive/Convert 4*uni8 to int2 ==
  byte0 : Inport
  byte1 : Inport  Port=2
  byte2 : Inport  Port=3
  byte3 : Inport  Port=4
  Add : Sum  Inputs=++++  OutDataTypeMode=int32  OutDataType=fixdt(1, 16)  OutScaling=2^-10  OutDataTypeStr=int32
  Gain2 : Gain  Gain=256  ParameterDataType=fixdt(1, 16)  ParameterScaling=2^0  OutDataType=fixdt(1, 16)  OutScaling=2^0
  Gain3 : Gain  Gain=2^16  ParameterDataType=fixdt(1, 16)  ParameterScaling=2^0  OutDataType=fixdt(1, 16)  OutScaling=2^0
  Gain4 : Gain  Gain=2^24  ParameterDataType=fixdt(1, 16)  ParameterScaling=2^0  OutDataType=fixdt(1, 16)  OutScaling=2^0
  int : Outport
  wires:
  Gain2/1 -> Add/2
  Gain3/1 -> Add/3
  byte0/1 -> Add/1
  Add/1 -> int/1
  byte1/1 -> Gain2/1
  byte2/1 -> Gain3/1
  byte3/1 -> Gain4/1
  Gain4/1 -> Add/4

== system Sim_Forcing_003h_expe_infra2/BEC (May 7, 2015)/CAN Receive/Convert 4*uni8 to int3 ==
  byte0 : Inport
  byte1 : Inport  Port=2
  byte2 : Inport  Port=3
  byte3 : Inport  Port=4
  Add : Sum  Inputs=++++  OutDataTypeMode=int32  OutDataType=fixdt(1, 16)  OutScaling=2^-10  OutDataTypeStr=int32
  Gain2 : Gain  Gain=256  ParameterDataType=fixdt(1, 16)  ParameterScaling=2^0  OutDataType=fixdt(1, 16)  OutScaling=2^0
  Gain3 : Gain  Gain=2^16  ParameterDataType=fixdt(1, 16)  ParameterScaling=2^0  OutDataType=fixdt(1, 16)  OutScaling=2^0
  Gain4 : Gain  Gain=2^24  ParameterDataType=fixdt(1, 16)  ParameterScaling=2^0  OutDataType=fixdt(1, 16)  OutScaling=2^0
  int : Outport
  wires:
  Gain4/1 -> Add/4
  byte3/1 -> Gain4/1
  byte2/1 -> Gain3/1
  byte1/1 -> Gain2/1
  Add/1 -> int/1
  byte0/1 -> Add/1
  Gain3/1 -> Add/3
  Gain2/1 -> Add/2

== system Sim_Forcing_003h_expe_infra2/BEC (May 7, 2015)/CAN Receive/Convert 4*uni8 to int4 ==
  byte0 : Inport
  byte1 : Inport  Port=2
  byte2 : Inport  Port=3
  byte3 : Inport  Port=4
  Add : Sum  Inputs=++++  OutDataTypeMode=int32  OutDataType=fixdt(1, 16)  OutScaling=2^-10  OutDataTypeStr=int32
  Gain2 : Gain  Gain=256  ParameterDataType=fixdt(1, 16)  ParameterScaling=2^0  OutDataType=fixdt(1, 16)  OutScaling=2^0
  Gain3 : Gain  Gain=2^16  ParameterDataType=fixdt(1, 16)  ParameterScaling=2^0  OutDataType=fixdt(1, 16)  OutScaling=2^0
  Gain4 : Gain  Gain=2^24  ParameterDataType=fixdt(1, 16)  ParameterScaling=2^0  OutDataType=fixdt(1, 16)  OutScaling=2^0
  int : Outport
  wires:
  Gain2/1 -> Add/2
  Gain3/1 -> Add/3
  byte0/1 -> Add/1
  Add/1 -> int/1
  byte1/1 -> Gain2/1
  byte2/1 -> Gain3/1
  byte3/1 -> Gain4/1
  Gain4/1 -> Add/4

== system Sim_Forcing_003h_expe_infra2/BEC (May 7, 2015)/CAN Receive/Convert 4*uni8 to int5 ==
  byte0 : Inport
  byte1 : Inport  Port=2
  byte2 : Inport  Port=3
  byte3 : Inport  Port=4
  Add : Sum  Inputs=++++  OutDataTypeMode=int32  OutDataType=fixdt(1, 16)  OutScaling=2^-10  OutDataTypeStr=int32
  Gain2 : Gain  Gain=256  ParameterDataType=fixdt(1, 16)  ParameterScaling=2^0  OutDataType=fixdt(1, 16)  OutScaling=2^0
  Gain3 : Gain  Gain=2^16  ParameterDataType=fixdt(1, 16)  ParameterScaling=2^0  OutDataType=fixdt(1, 16)  OutScaling=2^0
  Gain4 : Gain  Gain=2^24  ParameterDataType=fixdt(1, 16)  ParameterScaling=2^0  OutDataType=fixdt(1, 16)  OutScaling=2^0
  int : Outport
  wires:
  Gain4/1 -> Add/4
  byte3/1 -> Gain4/1
  byte2/1 -> Gain3/1
  byte1/1 -> Gain2/1
  Add/1 -> int/1
  byte0/1 -> Add/1
  Gain3/1 -> Add/3
  Gain2/1 -> Add/2

== system Sim_Forcing_003h_expe_infra2/BEC (May 7, 2015)/CAN Send/If Action Subsystem1 ==
  In1 : Inport  OutDataType=fixdt(1, 16)  OutScaling=2^0
  In2 : Inport  Port=2  OutDataType=fixdt(1, 16)  OutScaling=2^0
  In3 : Inport  Port=3  OutDataType=fixdt(1, 16)  OutScaling=2^0
  In4 : Inport  Port=4  OutDataType=fixdt(1, 16)  OutScaling=2^0
  In5 : Inport  Port=5  OutDataType=fixdt(1, 16)  OutScaling=2^0
  In6 : Inport  Port=6  OutDataType=fixdt(1, 16)  OutScaling=2^0
  Action Port : ActionPort  ActionType=then
  "Convert int to 4*uni8 " : Subsystem
  Convert int to 4*uni8 1 : Subsystem
  Convert int to 4*uni8 2 : Subsystem
  Convert int to 4*uni8 3 : Subsystem
  Convert int to 4*uni8 4 : Subsystem
  Convert int to 4*uni8 5 : Subsystem
  GT-RT CAN TX : gt_rt_lib/GT-RT CAN TX  uri='gt_rt_dev://localhost/dev/can0#0'  mff=MFF_11_DAT
  GT-RT CAN TX1 : gt_rt_lib/GT-RT CAN TX  uri='gt_rt_dev://localhost/dev/can0#0'  mff=MFF_11_DAT
  GT-RT CAN TX2 : gt_rt_lib/GT-RT CAN TX  uri='gt_rt_dev://localhost/dev/can0#0'  mff=MFF_11_DAT
  Mux : Mux  Inputs=2
  Mux1 : Mux  Inputs=2
  Mux2 : Mux  Inputs=2
  TX CAN ID1 : Constant  Value=hex2dec('101')  OutDataTypeMode=uint32  OutDataType=sfix(16)  OutScaling=2^0  OutDataTypeStr=uint32
  TX CAN ID2 : Constant  Value=hex2dec('102')  OutDataTypeMode=uint32  OutDataType=sfix(16)  OutScaling=2^0  OutDataTypeStr=uint32
  TX CAN ID3 : Constant  Value=hex2dec('103')  OutDataTypeMode=uint32  OutDataType=sfix(16)  OutScaling=2^0  OutDataTypeStr=uint32
  wires:
  In1/1 -> "Convert int to 4*uni8 "/1(in)
  In2/1 -> Convert int to 4*uni8 1/1(in)
  In3/1 -> Convert int to 4*uni8 2/1(in)
  In4/1 -> Convert int to 4*uni8 3/1(in)
  In5/1 -> Convert int to 4*uni8 4/1(in)
  In6/1 -> Convert int to 4*uni8 5/1(in)
  Mux2/1 -> GT-RT CAN TX2/2
  Convert int to 4*uni8 5/1(out) -> Mux2/2
  Convert int to 4*uni8 4/1(out) -> Mux2/1
  Mux1/1 -> GT-RT CAN TX1/2
  Convert int to 4*uni8 3/1(out) -> Mux1/2
  Convert int to 4*uni8 2/1(out) -> Mux1/1
  Mux/1 -> GT-RT CAN TX/2
  Convert int to 4*uni8 1/1(out) -> Mux/2
  "Convert int to 4*uni8 "/1(out) -> Mux/1
  TX CAN ID3/1 -> GT-RT CAN TX2/1
  TX CAN ID2/1 -> GT-RT CAN TX1/1
  TX CAN ID1/1 -> GT-RT CAN TX/1

== system Sim_Forcing_003h_expe_infra2/BEC (May 7, 2015)/Software limit switches/Subsystem ==
  In1 : Inport
  act : Inport  Port=2
  Abs1 : Abs  OutDataType=fixdt(1, 16)  OutScaling=2^0
  Abs2 : Abs  OutDataType=fixdt(1, 16)  OutScaling=2^0
  Add1 : Sum  Inputs=+-  OutDataType=fixdt(1, 16)  OutScaling=2^-10
  Add2 : Sum  Inputs=-+  OutDataType=fixdt(1, 16)  OutScaling=2^-10
  Display : Display
  Display2 : Display
  If Action Subsystem : Subsystem  TreatAsAtomicUnit=on
  If Action Subsystem1 : Subsystem  TreatAsAtomicUnit=on
  If2 : If
  NSEA1 : Constant  Value=-160  OutDataType=fixdt(1, 16)  OutScaling=2^0
  PSEA1 : Constant  Value=160  OutDataType=fixdt(1, 16)  OutScaling=2^0
  Switch : Switch  Criteria=u2 > Threshold  OutDataType=fixdt(1, 16)  OutScaling=2^0
  Switch1 : Switch  Criteria=u2 ~= 0  OutDataType=fixdt(1, 16)  OutScaling=2^0
  Out1 : Outport
  wires:
  If Action Subsystem1/1(Out1) -> Switch/3
  If Action Subsystem/1(Out1) -> Display/1, Switch/1
  Abs1/1 -> If Action Subsystem1/2(dif)
  If2/2 -> If Action Subsystem1/Action
  If2/1 -> If Action Subsystem/Action
  In1/1 -> If2/1, If Action Subsystem/2(Inc), If Action Subsystem1/1(Inc), Switch/2, Switch1/2, Switch1/3
  Abs2/1 -> If Action Subsystem/1(dif)
  NSEA1/1 -> Add1/2
  PSEA1/1 -> Add2/1
  Add1/1 -> Abs1/1
  Add2/1 -> Abs2/1
  Switch/1 -> Switch1/1
  Switch1/1 -> Out1/1, Display2/1
  act/1 -> Add1/1, Add2/2

== system Sim_Forcing_003h_expe_infra2/BEC (May 7, 2015)/Software limit switches/Subsystem1 ==
  In1 : Inport
  act : Inport  Port=2
  Abs1 : Abs  OutDataType=fixdt(1, 16)  OutScaling=2^0
  Abs2 : Abs  OutDataType=fixdt(1, 16)  OutScaling=2^0
  Add1 : Sum  Inputs=+-  OutDataType=fixdt(1, 16)  OutScaling=2^-10
  Add2 : Sum  Inputs=-+  OutDataType=fixdt(1, 16)  OutScaling=2^-10
  If Action Subsystem : Subsystem  TreatAsAtomicUnit=on
  If Action Subsystem1 : Subsystem  TreatAsAtomicUnit=on
  If2 : If
  NSEA1 : Constant  Value=-130  OutDataType=fixdt(1, 16)  OutScaling=2^0
  PSEA1 : Constant  Value=20  OutDataType=fixdt(1, 16)  OutScaling=2^0
  Switch : Switch  OutDataType=fixdt(1, 16)  OutScaling=2^0
  Switch1 : Switch  Criteria=u2 ~= 0  OutDataType=fixdt(1, 16)  OutScaling=2^0
  Out1 : Outport
  wires:
  act/1 -> Add1/1, Add2/2
  Add2/1 -> Abs2/1
  Add1/1 -> Abs1/1
  PSEA1/1 -> Add2/1
  NSEA1/1 -> Add1/2
  Abs2/1 -> If Action Subsystem/1(dif)
  In1/1 -> If Action Subsystem1/1(Inc), If Action Subsystem/2(Inc), Switch/2, Switch1/2, Switch1/3, If2/1
  If2/1 -> If Action Subsystem/Action
  If2/2 -> If Action Subsystem1/Action
  Abs1/1 -> If Action Subsystem1/2(dif)
  If Action Subsystem/1(Out1) -> Switch/1
  If Action Subsystem1/1(Out1) -> Switch/3
  Switch/1 -> Switch1/1
  Switch1/1 -> Out1/1

== system Sim_Forcing_003h_expe_infra2/BEC (May 7, 2015)/Software limit switches/Subsystem2 ==
  In1 : Inport
  act : Inport  Port=2
  Abs1 : Abs  OutDataType=fixdt(1, 16)  OutScaling=2^0
  Abs2 : Abs  OutDataType=fixdt(1, 16)  OutScaling=2^0
  Add1 : Sum  Inputs=+-  OutDataType=fixdt(1, 16)  OutScaling=2^-10
  Add2 : Sum  Inputs=-+  OutDataType=fixdt(1, 16)  OutScaling=2^-10
  If Action Subsystem : Subsystem  TreatAsAtomicUnit=on
  If Action Subsystem1 : Subsystem  TreatAsAtomicUnit=on
  If2 : If
  NSEA1 : Constant  Value=-88  OutDataType=fixdt(1, 16)  OutScaling=2^0
  PSEA1 : Constant  Value=88  OutDataType=fixdt(1, 16)  OutScaling=2^0
  Switch : Switch  OutDataType=fixdt(1, 16)  OutScaling=2^0
  Switch1 : Switch  Criteria=u2 ~= 0  OutDataType=fixdt(1, 16)  OutScaling=2^0
  Out1 : Outport
  wires:
  If Action Subsystem1/1(Out1) -> Switch/3
  If Action Subsystem/1(Out1) -> Switch/1
  Abs1/1 -> If Action Subsystem1/2(dif)
  If2/2 -> If Action Subsystem1/Action
  If2/1 -> If Action Subsystem/Action
  In1/1 -> If2/1, If Action Subsystem/2(Inc), If Action Subsystem1/1(Inc), Switch/2, Switch1/2, Switch1/3
  Abs2/1 -> If Action Subsystem/1(dif)
  NSEA1/1 -> Add1/2
  PSEA1/1 -> Add2/1
  Add1/1 -> Abs1/1
  Add2/1 -> Abs2/1
  act/1 -> Add1/1, Add2/2
  Switch/1 -> Switch1/1
  Switch1/1 -> Out1/1

== system Sim_Forcing_003h_expe_infra2/BEC (May 7, 2015)/Software limit switches/Subsystem3 ==
  In1 : Inport
  act : Inport  Port=2
  Abs1 : Abs  OutDataType=fixdt(1, 16)  OutScaling=2^0
  Abs2 : Abs  OutDataType=fixdt(1, 16)  OutScaling=2^0
  Add1 : Sum  Inputs=+-  OutDataType=fixdt(1, 16)  OutScaling=2^-10
  Add2 : Sum  Inputs=-+  OutDataType=fixdt(1, 16)  OutScaling=2^-10
  If Action Subsystem : Subsystem  TreatAsAtomicUnit=on
  If Action Subsystem1 : Subsystem  TreatAsAtomicUnit=on
  If2 : If
  NSEA1 : Constant  Value=-350  OutDataType=fixdt(1, 16)  OutScaling=2^0
  PSEA1 : Constant  Value=350  OutDataType=fixdt(1, 16)  OutScaling=2^0
  Switch : Switch  OutDataType=fixdt(1, 16)  OutScaling=2^0
  Switch1 : Switch  Criteria=u2 ~= 0  OutDataType=fixdt(1, 16)  OutScaling=2^0
  Out1 : Outport
  wires:
  Add2/1 -> Abs2/1
  Add1/1 -> Abs1/1
  PSEA1/1 -> Add2/1
  NSEA1/1 -> Add1/2
  Abs2/1 -> If Action Subsystem/1(dif)
  In1/1 -> If Action Subsystem1/1(Inc), If Action Subsystem/2(Inc), Switch/2, Switch1/2, Switch1/3, If2/1
  If2/1 -> If Action Subsystem/Action
  If2/2 -> If Action Subsystem1/Action
  act/1 -> Add2/2, Add1/1
  Abs1/1 -> If Action Subsystem1/2(dif)
  If Action Subsystem/1(Out1) -> Switch/1
  If Action Subsystem1/1(Out1) -> Switch/3
  Switch/1 -> Switch1/1
  Switch1/1 -> Out1/1

== system Sim_Forcing_003h_expe_infra2/BEC (May 7, 2015)/Software limit switches/Subsystem4 ==
  In1 : Inport
  act : Inport  Port=2
  Abs1 : Abs  OutDataType=fixdt(1, 16)  OutScaling=2^0
  Abs2 : Abs  OutDataType=fixdt(1, 16)  OutScaling=2^0
  Add1 : Sum  Inputs=+-  OutDataType=fixdt(1, 16)  OutScaling=2^-10
  Add2 : Sum  Inputs=-+  OutDataType=fixdt(1, 16)  OutScaling=2^-10
  If Action Subsystem : Subsystem  TreatAsAtomicUnit=on
  If Action Subsystem1 : Subsystem  TreatAsAtomicUnit=on
  If2 : If
  NSEA1 : Constant  Value=-61  OutDataType=fixdt(1, 16)  OutScaling=2^0
  PSEA1 : Constant  Value=61  OutDataType=fixdt(1, 16)  OutScaling=2^0
  Switch : Switch  OutDataType=fixdt(1, 16)  OutScaling=2^0
  Switch1 : Switch  Criteria=u2 ~= 0  OutDataType=fixdt(1, 16)  OutScaling=2^0
  Out1 : Outport
  wires:
  If Action Subsystem/1(Out1) -> Switch/1
  Abs1/1 -> If Action Subsystem1/2(dif)
  If2/2 -> If Action Subsystem1/Action
  If2/1 -> If Action Subsystem/Action
  In1/1 -> If2/1, If Action Subsystem/2(Inc), If Action Subsystem1/1(Inc), Switch/2, Switch1/2, Switch1/3
  Abs2/1 -> If Action Subsystem/1(dif)
  NSEA1/1 -> Add1/2
  PSEA1/1 -> Add2/1
  Add1/1 -> Abs1/1
  Add2/1 -> Abs2/1
  If Action Subsystem1/1(Out1) -> Switch/3
  Switch/1 -> Switch1/1
  Switch1/1 -> Out1/1
  act/1 -> Add2/2, Add1/1

== system Sim_Forcing_003h_expe_infra2/BEC (May 7, 2015)/Software limit switches/Subsystem5 ==
  In1 : Inport
  act : Inport  Port=2
  Abs1 : Abs  OutDataType=fixdt(1, 16)  OutScaling=2^0
  Abs2 : Abs  OutDataType=fixdt(1, 16)  OutScaling=2^0
  Add1 : Sum  Inputs=+-  OutDataType=fixdt(1, 16)  OutScaling=2^-10
  Add2 : Sum  Inputs=-+  OutDataType=fixdt(1, 16)  OutScaling=2^-10
  If Action Subsystem : Subsystem  TreatAsAtomicUnit=on
  If Action Subsystem1 : Subsystem  TreatAsAtomicUnit=on
  If2 : If
  NSEA1 : Constant  Value=-350  OutDataType=fixdt(1, 16)  OutScaling=2^0
  PSEA1 : Constant  Value=350  OutDataType=fixdt(1, 16)  OutScaling=2^0
  Switch : Switch  OutDataType=fixdt(1, 16)  OutScaling=2^0
  Switch1 : Switch  Criteria=u2 ~= 0  OutDataType=fixdt(1, 16)  OutScaling=2^0
  Out1 : Outport
  wires:
  Add2/1 -> Abs2/1
  Add1/1 -> Abs1/1
  PSEA1/1 -> Add2/1
  NSEA1/1 -> Add1/2
  Abs2/1 -> If Action Subsystem/1(dif)
  In1/1 -> If Action Subsystem1/1(Inc), If Action Subsystem/2(Inc), Switch/2, Switch1/2, Switch1/3, If2/1
  If2/1 -> If Action Subsystem/Action
  If2/2 -> If Action Subsystem1/Action
  Abs1/1 -> If Action Subsystem1/2(dif)
  If Action Subsystem/1(Out1) -> Switch/1
  If Action Subsystem1/1(Out1) -> Switch/3
  Switch/1 -> Switch1/1
  Switch1/1 -> Out1/1
  act/1 -> Add2/2, Add1/1
